simulink model "Threephase_inverter"  (R2020a)
settings: Solver=VariableStepAuto  StartTime=0.0  StopTime=0.0334  RelTol=1e-3
libraries: powerlib x13
settings Model: Creator=Naeem Mohammad  LastModifiedBy=Naeem Mohammad

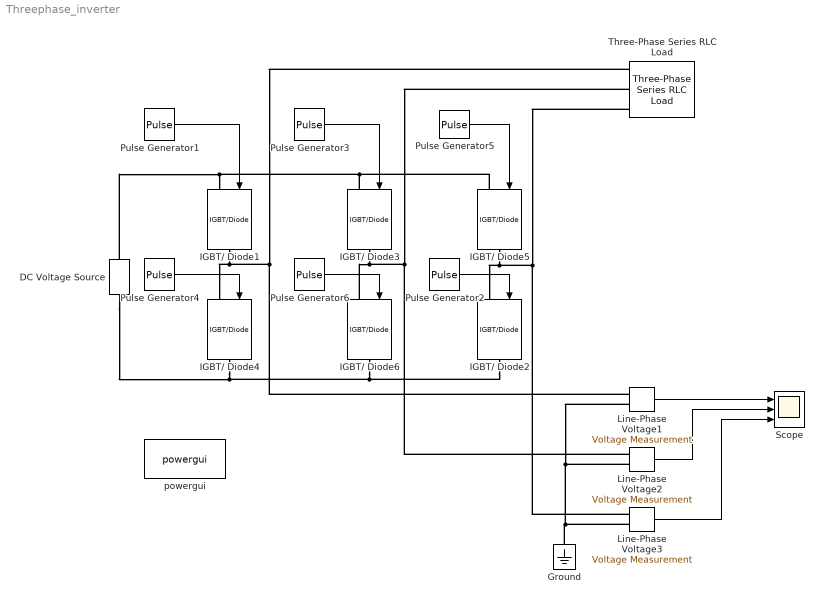
== system Threephase_inverter ==
  DC Voltage Source : powerlib/Electrical Sources/DC Voltage Source  Amplitude=48  Measurements=None
  Ground : powerlib/Elements/Ground  LConnTagsString=a
  IGBT/ Diode{1..6} (6 alike) : powerlib/Power Electronics/IGBT//Diode  Ron=1e-3  Rs=1e5  Cs=inf  Measurements=off
  Line-Phase Voltage1 : powerlib/Measurements/Voltage Measurement  PhasorSimulation=off  OutputType=Complex  PSBequivalent=0
  Line-Phase Voltage2 : powerlib/Measurements/Voltage Measurement  PhasorSimulation=off  OutputType=Complex  PSBequivalent=0
  Line-Phase Voltage3 : powerlib/Measurements/Voltage Measurement  PhasorSimulation=off  OutputType=Complex  PSBequivalent=0
  Pulse Generator1 : DiscretePulseGenerator  PulseType=Time based  Period=1/60  PulseWidth=50
  Pulse Generator2 : DiscretePulseGenerator  PulseType=Time based  Period=1/60  PulseWidth=50  PhaseDelay=60*(1/60)*(1/360)
  Pulse Generator3 : DiscretePulseGenerator  PulseType=Time based  Period=1/60  PulseWidth=50  PhaseDelay=120*(1/60)*(1/360)
  Pulse Generator4 : DiscretePulseGenerator  PulseType=Time based  Period=1/60  PulseWidth=50  PhaseDelay=180*(1/60)*(1/360)
  Pulse Generator5 : DiscretePulseGenerator  PulseType=Time based  Period=1/60  PulseWidth=50  PhaseDelay=240*(1/60)*(1/360)
  Pulse Generator6 : DiscretePulseGenerator  PulseType=Time based  Period=1/60  PulseWidth=50  PhaseDelay=300*(1/60)*(1/360)
  Scope : Scope  NumInputPorts=3
  Three-Phase Series RLC Load : powerlib/Elements/Three-Phase Series RLC Load  LConnTagsString=A|B|C  Configuration=Y (grounded)  NominalVoltage=1000  Vabc=[1e3 1e3 1e3]  Vabcp=[1e3 1e3 1e3]  NominalFrequency=60  UnbalancedPower=off  ActivePower=10e3  InductivePower=100  CapacitivePower=100  Pabc=[10e3 9e3 11e3]  QLabc=[100 90 110]  QCabc=[100 90 110]  Pabcp=[10e3 9e3 11e3]  QLabcp=[100 90 110]  QCabcp=[100 90 110]  Measurements=None  LoadType=constant Z
  powergui : powerlib/powergui  Priority=1  SimulationMode=Continuous  SampleTime=50e-6  frequency=60  Iterations=50  frequencyindice=0  Pbase=100e6  ErrMax=1e-4  UnitsV=kV  UnitsW=MW  buscounter=0  FunctionMessages=off  echomessages=off  EnableUseOfTLC=off  CurrentSourceSwitches=off  DisableSnubberDevices=off  DisableRonSwitches=off  DisableVfSwitches=off  DisplayEquations=off  AutomaticDiscreteSolvers=off  SolverType=Tustin/Backward Euler (TBE)  Interpol=off  ExternalGateDelay=off  methode=off  Ts=100  x0status=blocks  SPID=on  SwTol=0  HookPort=off  NonlinearTolerance=1e-4  nMaxIteration=100  ContinueOnMaxIteration=off  RestoreLinks=warning  ResistiveCurrentMeasurement=off  Frange=[0:2:500]  Ylog=off  Xlog=on  ShowGrid=off  save=off  variable=ZData  structure=0  ZoomFFT=off  StartTime=0.0  cycles=1  DisplayStyle=1  fundamental=60  FreqAxis=off  MaxFrequency=1000  frequencyindicesteady=1  RmsSteady=1  display=off
  wires:
  Pulse Generator1/1 -> IGBT/ Diode1/1
  Pulse Generator3/1 -> IGBT/ Diode3/1
  Line-Phase Voltage1/1 -> Scope/1
  Line-Phase Voltage2/1 -> Scope/2
  Line-Phase Voltage3/1 -> Scope/3
  Pulse Generator4/1 -> IGBT/ Diode4/1
  Pulse Generator5/1 -> IGBT/ Diode5/1
  Pulse Generator6/1 -> IGBT/ Diode6/1
  Pulse Generator2/1 -> IGBT/ Diode2/1
  connections:
  IGBT/ Diode1/RConn1 -- Three-Phase Series RLC Load/LConn1 -- Line-Phase Voltage1/LConn1 -- IGBT/ Diode4/LConn1
  DC Voltage Source/RConn1 -- IGBT/ Diode5/LConn1 -- IGBT/ Diode3/LConn1 -- IGBT/ Diode1/LConn1
  DC Voltage Source/LConn1 -- IGBT/ Diode4/RConn1 -- IGBT/ Diode2/RConn1 -- IGBT/ Diode6/RConn1
  IGBT/ Diode3/RConn1 -- IGBT/ Diode6/LConn1 -- Line-Phase Voltage2/LConn1 -- Three-Phase Series RLC Load/LConn2
  Line-Phase Voltage3/LConn1 -- Three-Phase Series RLC Load/LConn3 -- IGBT/ Diode5/RConn1 -- IGBT/ Diode2/LConn1
  Line-Phase Voltage2/LConn2 -- Line-Phase Voltage3/LConn2 -- Ground/LConn1 -- Line-Phase Voltage1/LConn2
